simulink model "basic_complementary_filter_for_pixhawk"  (R2021b)
settings: Solver=FixedStepAuto  StartTime=0.0  StopTime=inf  RelTol=1e-3  EnableMultiTasking=on
undefined symbols (not defined in the file): DiscIntNeverNeededParam
libraries: simulink_extras x9, px4Sensorslib x3
settings Model: SimulationMode=external  ExtModeTrigDuration=10  Creator=asus  LastModifiedBy=Burhan
settings SolverCC: AlgebraicLoopSolver=TrustRegion  PositivePriorityOrder=on
settings OptimizationCC: EnhancedBackFolding=on  PassReuseOutputArgsAs=Individual arguments  MaxStackSize=64  OptimizeBlockOrder=speed  DifferentSizesBufferReuse=on  OptimizationCustomize=off  EfficientTunableParamExpr=on
settings DebuggingCC: ParameterTunabilityLossMsg=error  SFMachineParentedDataDiag=warning
settings HardwareCC: ProdBitPerPointer=32  ProdBitPerSizeT=32  ProdBitPerPtrDiffT=32  ProdLargestAtomicInteger=Long  ProdLargestAtomicFloat=Double  ProdWordSize=32  ProdLongLongMode=on  ProdHWDeviceType=ARM Compatible->ARM Cortex
settings SFSimCC: MATLABDynamicMemAlloc=off  CustomCodeUndefinedFunction=UseInterfaceOnly  SimTargetLang=C++
settings RTWCC: Description=Embedded Coder  SystemTargetFile=ert.tlc  HardwareBoard=PX4 Pixhawk Series  TLCOptions="-aInlineSetEventsForThisBaseRateFcn=TLC_FALSE -aSuppressMultiTaskScheduler=TLC_FALSE  -aRateBasedStepFcn=0"  TemplateMakefile=ert_default_tmf  GenerateReport=on  Toolchain=GNU Tools for PX4 Autopilots  IncludeHyperlinkInReport=on  LaunchReport=on  TargetLang=C++  GenerateTraceInfo=on  GenerateTraceReport=on  GenerateTraceReportSl=on  GenerateTraceReportSf=on  GenerateTraceReportEml=on
settings CodeAppCC: ForceParamTrailComments=on  IgnoreCustomStorageClasses=off  OperatorAnnotations=on  SimulinkDataObjDesc=on  SFDataObjDesc=on  InsertBlockDesc=on

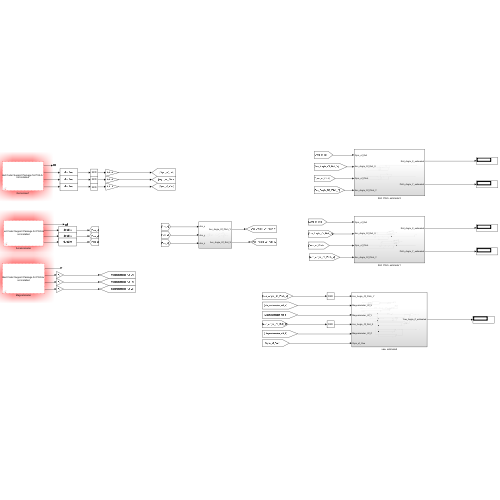
[thumbnail: Simulink's stored preview of the top-level diagram]
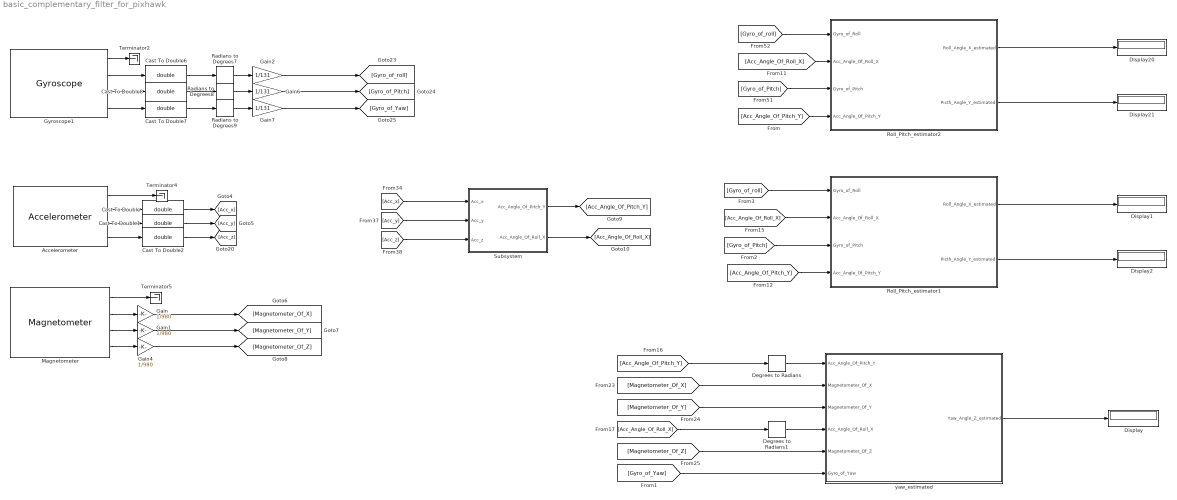
== system basic_complementary_filter_for_pixhawk ==
  Accelerometer : px4Sensorslib/Accelerometer  uorbTimeStamp=off  BlockingMode=off  BlockTimeout=1e-3  sampleTime=0.1
      settings: SourceProductName=Embedded Coder Support Package for PX4 Autopilots
  Cast To Double{,1..2,6..8} (6 alike) : DataTypeConversion  OutDataTypeStr=double
  Degrees to Radians : simulink_extras/Transformations/Degrees to Radians
  Degrees to Radians1 : simulink_extras/Transformations/Degrees to Radians
  Display{,1..2,20..21} (5 alike) : Display
  Gain : Gain  Gain=1/980
  Gain1 : Gain  Gain=1/980
  Gain2 : Gain  Gain=1/131
  Gain4 : Gain  Gain=1/980
  Gain6 : Gain  Gain=1/131
  Gain7 : Gain  Gain=1/131
  Gyroscope1 : px4Sensorslib/Gyroscope  uorbTimeStamp=off  BlockingMode=off  BlockTimeout=1e-3  sampleTime=-1
      settings: SourceProductName=Embedded Coder Support Package for PX4 Autopilots
  Magnetometer : px4Sensorslib/Magnetometer  uorbTimeStamp=off  BlockingMode=off  BlockTimeout=1e-3  sampleTime=0.1
      settings: SourceProductName=Embedded Coder Support Package for PX4 Autopilots
  Radians to Degrees7 : simulink_extras/Transformations/Radians to Degrees
  Radians to Degrees8 : simulink_extras/Transformations/Radians to Degrees
  Radians to Degrees9 : simulink_extras/Transformations/Radians to Degrees
  Roll_Pitch_estimator1 : Subsystem
  Roll_Pitch_estimator2 : Subsystem
  Subsystem : Subsystem
  Terminator2 : Terminator
  Terminator4 : Terminator
  Terminator5 : Terminator
  yaw_estimated : Subsystem
  wires:
  Cast To Double/1 -> [Acc_x]
  Accelerometer/1 -> Terminator4/1
  Accelerometer/4 -> Cast To Double2/1
  Accelerometer/2 -> Cast To Double/1
  Cast To Double6/1 -> Radians to Degrees7/1
  [Acc_Angle_Of_Pitch_Y] -> Roll_Pitch_estimator2/4(Acc_Angle_Of_Pitch_Y)
  Cast To Double7/1 -> Radians to Degrees9/1
  Roll_Pitch_estimator2/1(Roll_Angle_X_estimated) -> Display20/1
  [Gyro_of_Pitch] -> Roll_Pitch_estimator2/3(Gyro_of_Pitch)
  Gyroscope1/2 -> Cast To Double6/1
  Gyroscope1/1 -> Terminator2/1
  Gyroscope1/4 -> Cast To Double7/1
  Gain6/1 -> [Gyro_of_Pitch]
  Roll_Pitch_estimator2/2(Picth_Angle_Y_estimated) -> Display21/1
  Cast To Double1/1 -> [Acc_y]
  Accelerometer/3 -> Cast To Double1/1
  Cast To Double8/1 -> Radians to Degrees8/1
  Radians to Degrees8/1 -> Gain6/1
  Radians to Degrees7/1 -> Gain2/1
  Gyroscope1/3 -> Cast To Double8/1
  Gain7/1 -> [Gyro_of_Yaw]
  [Acc_Angle_Of_Roll_X] -> Roll_Pitch_estimator2/2(Acc_Angle_Of_Roll_X)
  Gain2/1 -> [Gyro_of_roll]
  Radians to Degrees9/1 -> Gain7/1
  [Gyro_of_roll] -> Roll_Pitch_estimator2/1(Gyro_of_Roll)
  [Gyro_of_roll] -> Roll_Pitch_estimator1/1(Gyro_of_Roll)
  [Acc_Angle_Of_Roll_X] -> Roll_Pitch_estimator1/2(Acc_Angle_Of_Roll_X)
  Roll_Pitch_estimator1/2(Picth_Angle_Y_estimated) -> Display2/1
  [Gyro_of_Pitch] -> Roll_Pitch_estimator1/3(Gyro_of_Pitch)
  Roll_Pitch_estimator1/1(Roll_Angle_X_estimated) -> Display1/1
  [Acc_Angle_Of_Pitch_Y] -> Roll_Pitch_estimator1/4(Acc_Angle_Of_Pitch_Y)
  [Acc_Angle_Of_Roll_X] -> Degrees to Radians1/1
  [Magnetometer_Of_X] -> yaw_estimated/2(Magnetometer_Of_X)
  [Magnetometer_Of_Y] -> yaw_estimated/3(Magnetometer_Of_Y)
  [Gyro_of_Yaw] -> yaw_estimated/6(Gyro_of_Yaw)
  yaw_estimated/1(Yaw_Angle_Z_estimated) -> Display/1
  [Acc_Angle_Of_Pitch_Y] -> Degrees to Radians/1
  [Magnetometer_Of_Z] -> yaw_estimated/5(Magnetometer_Of_Z)
  Magnetometer/3 -> Gain1/1
  Magnetometer/1 -> Terminator5/1
  Magnetometer/2 -> Gain/1
  Degrees to Radians/1 -> yaw_estimated/1(Acc_Angle_Of_Pitch_Y)
  Degrees to Radians1/1 -> yaw_estimated/4(Acc_Angle_Of_Roll_X)
  Cast To Double2/1 -> [Acc_z]
  Gain/1 -> [Magnetometer_Of_X]
  Gain1/1 -> [Magnetometer_Of_Y]
  Magnetometer/4 -> Gain4/1
  Gain4/1 -> [Magnetometer_Of_Z]
  [Acc_x] -> Subsystem/1(Acc_x)
  [Acc_y] -> Subsystem/2(Acc_y)
  [Acc_z] -> Subsystem/3(Acc_z)
  Subsystem/1(Acc_Angle_Of_Pitch_Y) -> [Acc_Angle_Of_Pitch_Y]
  Subsystem/2(Acc_Angle_Of_Roll_X) -> [Acc_Angle_Of_Roll_X]

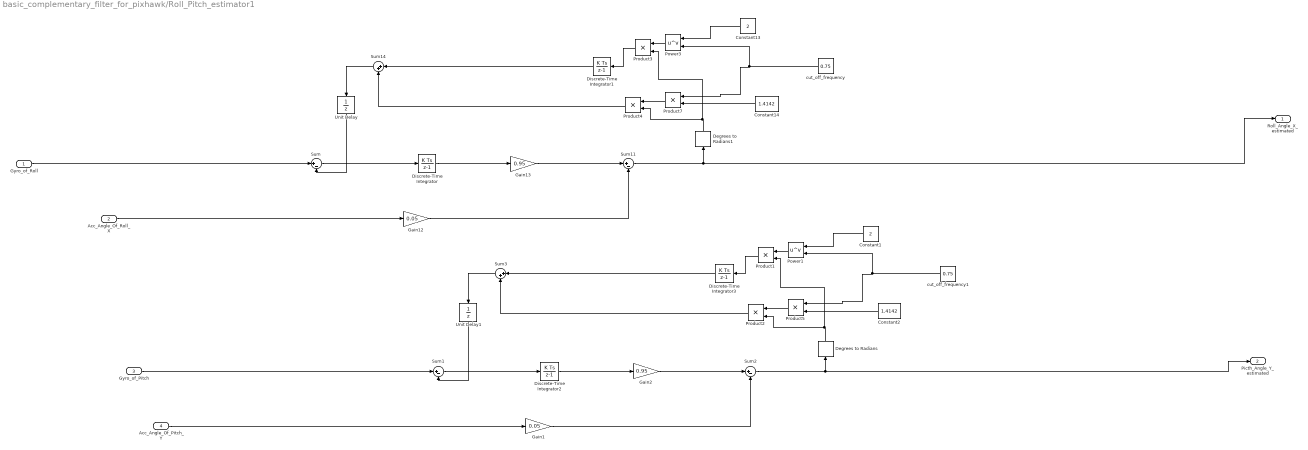
== system basic_complementary_filter_for_pixhawk/Roll_Pitch_estimator1 ==
  Gyro_of_Roll : Inport
  Acc_Angle_Of_Roll_X : Inport  Port=2
  Gyro_of_Pitch : Inport  Port=3
  Acc_Angle_Of_Pitch_Y : Inport  Port=4
  Constant1 : Constant  Value=2
  Constant13 : Constant  Value=2
  Constant14 : Constant  Value=1.4142
  Constant2 : Constant  Value=1.4142
  Degrees to Radians : simulink_extras/Transformations/Degrees to Radians
  Degrees to Radians1 : simulink_extras/Transformations/Degrees to Radians
  Discrete-Time Integrator{,1..3} (4 alike) : DiscreteIntegrator  SampleTime=-1  ICPrevOutput=DiscIntNeverNeededParam  ICPrevScaledInput=DiscIntNeverNeededParam
  Gain1 : Gain  Gain=0.05
  Gain12 : Gain  Gain=0.05
  Gain13 : Gain  Gain=0.95
  Gain2 : Gain  Gain=0.95
  Power1 : Math  Operator=pow  SignedPower=on  SaturateOnIntegerOverflow=on
  Power3 : Math  Operator=pow  SignedPower=on  SaturateOnIntegerOverflow=on
  Product{1..5,7} (6 alike) : Product
  Sum{,1..2,11} (4 alike) : Sum  Inputs=|+-
  Sum14 : Sum  Inputs=|++
  Sum3 : Sum  Inputs=|++
  Unit Delay : UnitDelay  SampleTime=-1  HasFrameUpgradeWarning=on
  Unit Delay1 : UnitDelay  SampleTime=-1  HasFrameUpgradeWarning=on
  cut_off_frequency : Constant  Value=0.75
  cut_off_frequency1 : Constant  Value=0.75
  Roll_Angle_X_estimated : Outport  VectorParamsAs1DForOutWhenUnconnected=off
  Picth_Angle_Y_estimated : Outport  Port=2  VectorParamsAs1DForOutWhenUnconnected=off
  wires:
  Discrete-Time Integrator/1 -> Gain13/1
  Acc_Angle_Of_Roll_X/1 -> Gain12/1
  Gain13/1 -> Sum11/1
  Gain12/1 -> Sum11/2
  Constant13/1 -> Power3/1
  Sum14/1 -> Unit Delay/1
  Unit Delay/1 -> Sum/2
  Discrete-Time Integrator1/1 -> Sum14/1
  Power3/1 -> Product3/1
  Constant14/1 -> Product7/2
  Product3/1 -> Discrete-Time Integrator1/1
  Product4/1 -> Sum14/2
  Product7/1 -> Product4/1
  Sum11/1 -> Degrees to Radians1/1, Roll_Angle_X_estimated/1
  Gyro_of_Roll/1 -> Sum/1
  Sum/1 -> Discrete-Time Integrator/1
  cut_off_frequency/1 -> Power3/2, Product7/1
  cut_off_frequency1/1 -> Product5/1, Power1/2
  Sum1/1 -> Discrete-Time Integrator2/1
  Gyro_of_Pitch/1 -> Sum1/1
  Sum2/1 -> Degrees to Radians/1, Picth_Angle_Y_estimated/1
  Product5/1 -> Product2/1
  Product2/1 -> Sum3/2
  Product1/1 -> Discrete-Time Integrator3/1
  Constant2/1 -> Product5/2
  Power1/1 -> Product1/1
  Discrete-Time Integrator3/1 -> Sum3/1
  Unit Delay1/1 -> Sum1/2
  Sum3/1 -> Unit Delay1/1
  Constant1/1 -> Power1/1
  Gain1/1 -> Sum2/2
  Gain2/1 -> Sum2/1
  Acc_Angle_Of_Pitch_Y/1 -> Gain1/1
  Discrete-Time Integrator2/1 -> Gain2/1
  Degrees to Radians/1 -> Product2/2, Product1/2
  Degrees to Radians1/1 -> Product3/2, Product4/2

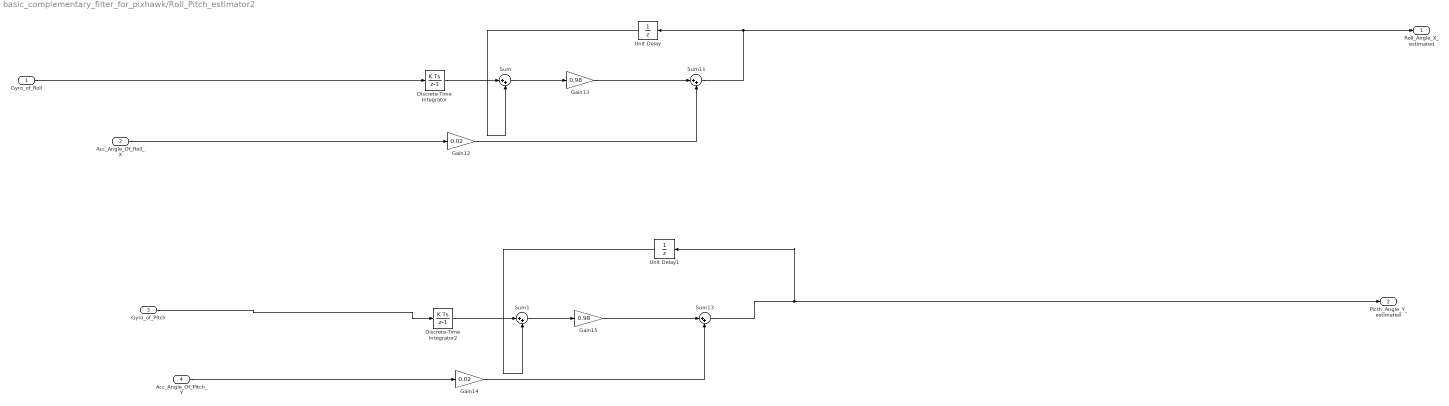
== system basic_complementary_filter_for_pixhawk/Roll_Pitch_estimator2 ==
  Gyro_of_Roll : Inport
  Acc_Angle_Of_Roll_X : Inport  Port=2
  Gyro_of_Pitch : Inport  Port=3
  Acc_Angle_Of_Pitch_Y : Inport  Port=4
  Discrete-Time Integrator : DiscreteIntegrator  SampleTime=-1  ICPrevOutput=DiscIntNeverNeededParam  ICPrevScaledInput=DiscIntNeverNeededParam
  Discrete-Time Integrator2 : DiscreteIntegrator  SampleTime=-1  ICPrevOutput=DiscIntNeverNeededParam  ICPrevScaledInput=DiscIntNeverNeededParam
  Gain12 : Gain  Gain=0.02
  Gain13 : Gain  Gain=0.98
  Gain14 : Gain  Gain=0.02
  Gain15 : Gain  Gain=0.98
  Sum{,1,11,13} (4 alike) : Sum  Inputs=|++
  Unit Delay : UnitDelay  SampleTime=-1  HasFrameUpgradeWarning=on
  Unit Delay1 : UnitDelay  SampleTime=-1  HasFrameUpgradeWarning=on
  Roll_Angle_X_estimated : Outport  VectorParamsAs1DForOutWhenUnconnected=off
  Picth_Angle_Y_estimated : Outport  Port=2  VectorParamsAs1DForOutWhenUnconnected=off
  wires:
  Sum11/1 -> Roll_Angle_X_estimated/1, Unit Delay/1
  Gyro_of_Roll/1 -> Discrete-Time Integrator/1
  Gyro_of_Pitch/1 -> Discrete-Time Integrator2/1
  Gain15/1 -> Sum13/1
  Gain12/1 -> Sum11/2
  Gain14/1 -> Sum13/2
  Gain13/1 -> Sum11/1
  Acc_Angle_Of_Pitch_Y/1 -> Gain14/1
  Sum13/1 -> Unit Delay1/1, Picth_Angle_Y_estimated/1
  Acc_Angle_Of_Roll_X/1 -> Gain12/1
  Discrete-Time Integrator/1 -> Sum/1
  Sum/1 -> Gain13/1
  Sum1/1 -> Gain15/1
  Discrete-Time Integrator2/1 -> Sum1/1
  Unit Delay/1 -> Sum/2
  Unit Delay1/1 -> Sum1/2

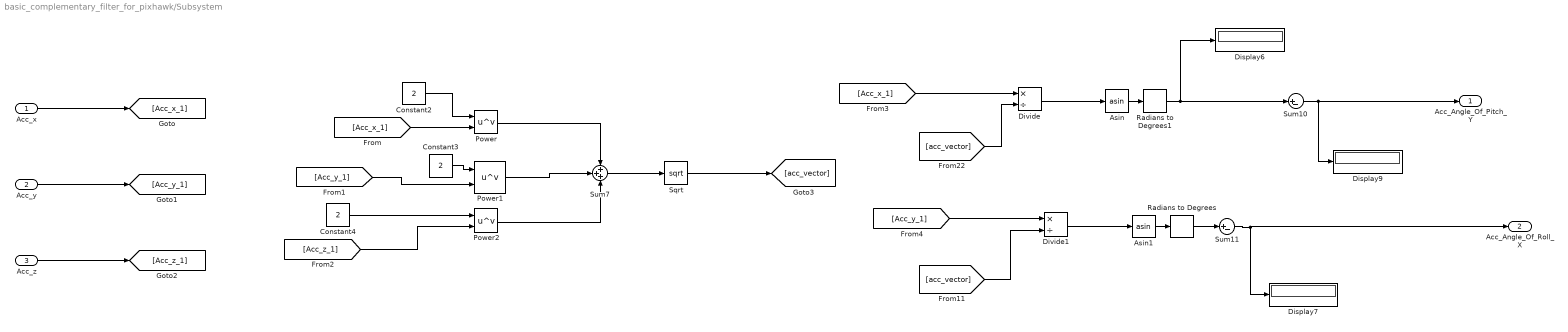
== system basic_complementary_filter_for_pixhawk/Subsystem ==
  Acc_x : Inport
  Acc_y : Inport  Port=2
  Acc_z : Inport  Port=3
  Asin : Trigonometry  Operator=asin
  Asin1 : Trigonometry  Operator=asin
  Constant2 : Constant  Value=2
  Constant3 : Constant  Value=2
  Constant4 : Constant  Value=2
  Display6 : Display
      settings: Decimation=3
  Display7 : Display
  Display9 : Display
  Divide : Product  Inputs=*/
  Divide1 : Product  Inputs=*/
  Power : Math  Operator=pow  SignedPower=on  SaturateOnIntegerOverflow=on
  Power1 : Math  Operator=pow  SignedPower=on  SaturateOnIntegerOverflow=on
  Power2 : Math  Operator=pow  SignedPower=on  SaturateOnIntegerOverflow=on
  Radians to Degrees : simulink_extras/Transformations/Radians to Degrees
  Radians to Degrees1 : simulink_extras/Transformations/Radians to Degrees
  Sqrt : Sqrt  SaturateOnIntegerOverflow=on
  Sum10 : Sum  Inputs=|+-
  Sum11 : Sum  Inputs=|+-
  Sum7 : Sum  Inputs=+++
  Acc_Angle_Of_Pitch_Y : Outport  VectorParamsAs1DForOutWhenUnconnected=off
  Acc_Angle_Of_Roll_X : Outport  Port=2  VectorParamsAs1DForOutWhenUnconnected=off
  wires:
  Divide1/1 -> Asin1/1
  Asin/1 -> Radians to Degrees1/1
  Divide/1 -> Asin/1
  Constant3/1 -> Power1/1
  Sum10/1 -> Acc_Angle_Of_Pitch_Y/1, Display9/1
  Power1/1 -> Sum7/2
  Asin1/1 -> Radians to Degrees/1
  Power/1 -> Sum7/1
  [acc_vector] -> Divide/2
  Radians to Degrees1/1 -> Sum10/1, Display6/1
  Radians to Degrees/1 -> Sum11/1
  Power2/1 -> Sum7/3
  Constant4/1 -> Power2/1
  Constant2/1 -> Power/1
  [acc_vector] -> Divide1/2
  Sqrt/1 -> [acc_vector]
  Sum11/1 -> Acc_Angle_Of_Roll_X/1, Display7/1
  [Acc_x_1] -> Divide/1
  [Acc_y_1] -> Divide1/1
  Sum7/1 -> Sqrt/1
  Acc_x/1 -> [Acc_x_1]
  Acc_y/1 -> [Acc_y_1]
  Acc_z/1 -> [Acc_z_1]
  [Acc_x_1] -> Power/2
  [Acc_y_1] -> Power1/2
  [Acc_z_1] -> Power2/2

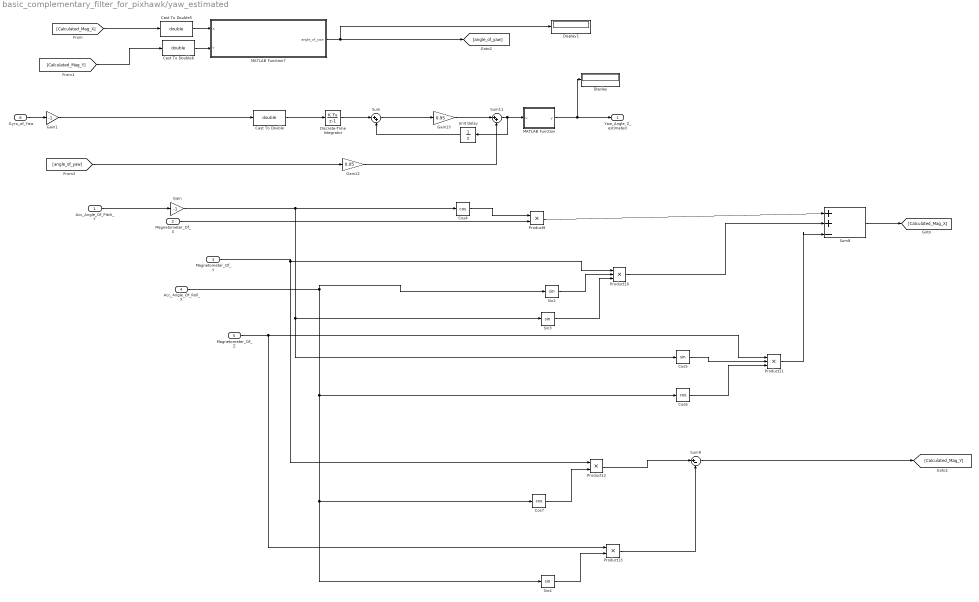
== system basic_complementary_filter_for_pixhawk/yaw_estimated ==
  Acc_Angle_Of_Pitch_Y : Inport
  Magnetometer_Of_X : Inport  Port=2
  Magnetometer_Of_Y : Inport  Port=3
  Acc_Angle_Of_Roll_X : Inport  Port=4
  Magnetometer_Of_Z : Inport  Port=5
  Gyro_of_Yaw : Inport  Port=6
  Cast To Double : DataTypeConversion  OutDataTypeStr=double
  Cast To Double5 : DataTypeConversion  OutDataTypeStr=double
  Cast To Double6 : DataTypeConversion  OutDataTypeStr=double
  Cos4 : Trigonometry  Operator=cos
  Cos5 : Trigonometry
  Cos6 : Trigonometry  Operator=cos
  Cos7 : Trigonometry  Operator=cos
  Discrete-Time Integrator : DiscreteIntegrator  SampleTime=-1  ICPrevOutput=DiscIntNeverNeededParam  ICPrevScaledInput=DiscIntNeverNeededParam
  Display : Display
  Display1 : Display
  Gain : Gain  Gain=-1
  Gain1 : Gain  Gain=-1
  Gain12 : Gain  Gain=0.05
  Gain13 : Gain  Gain=0.95
  MATLAB Function : MATLAB Function  TreatAsAtomicUnit=on
  MATLAB Function7 : MATLAB Function  TreatAsAtomicUnit=on
  Product10 : Product  Inputs=3
  Product11 : Product  Inputs=3
  Product12 : Product
  Product13 : Product
  Product9 : Product
  Sin2 : Trigonometry
  Sin3 : Trigonometry
  Sin4 : Trigonometry
  Sum : Sum  Inputs=|++
  Sum11 : Sum  Inputs=|++
  Sum8 : Sum  Inputs=|++-
  Sum9 : Sum  Inputs=|+-
  Unit Delay : UnitDelay  SampleTime=-1  HasFrameUpgradeWarning=on
  Yaw_Angle_Z_estimated : Outport  VectorParamsAs1DForOutWhenUnconnected=off
  wires:
  Acc_Angle_Of_Roll_X/1 -> Sin4/1, Cos7/1, Cos6/1, Sin2/1
  Cos6/1 -> Product11/3
  Product11/1 -> Sum8/3
  [Calculated_Mag_X] -> Cast To Double5/1
  Acc_Angle_Of_Pitch_Y/1 -> Gain/1
  Magnetometer_Of_X/1 -> Product9/2
  Magnetometer_Of_Y/1 -> Product12/1, Product10/1
  Sin2/1 -> Product10/2
  Product12/1 -> Sum9/1
  Sin3/1 -> Product10/3
  Cos7/1 -> Product12/2
  Cos5/1 -> Product11/2
  Sin4/1 -> Product13/2
  Product9/1 -> Sum8/1
  Product10/1 -> Sum8/2
  Cast To Double5/1 -> MATLAB Function7/1(X)
  Product13/1 -> Sum9/2
  Magnetometer_Of_Z/1 -> Product13/1, Product11/1
  Cast To Double6/1 -> MATLAB Function7/2(Y)
  [Calculated_Mag_Y] -> Cast To Double6/1
  Sum9/1 -> [Calculated_Mag_Y]
  Cos4/1 -> Product9/1
  Sum8/1 -> [Calculated_Mag_X]
  [angle_of_yaw] -> Gain12/1
  Gyro_of_Yaw/1 -> Gain1/1
  Cast To Double/1 -> Discrete-Time Integrator/1
  Gain12/1 -> Sum11/2
  Gain13/1 -> Sum11/1
  Sum11/1 -> Unit Delay/1, MATLAB Function/1(u)
  MATLAB Function7/1(angle_of_yaw) -> Display1/1, [angle_of_yaw]
  Discrete-Time Integrator/1 -> Sum/1
  Sum/1 -> Gain13/1
  Unit Delay/1 -> Sum/2
  Gain/1 -> Cos5/1, Sin3/1, Cos4/1
  Gain1/1 -> Cast To Double/1
  MATLAB Function/1(y) -> Display/1, Yaw_Angle_Z_estimated/1

== matlab function basic_complementary_filter_for_pixhawk/yaw_estimated/MATLAB Function7 ==
  data: X input; angle_of_yaw output; Y input
function angle_of_yaw = fcn(X, Y)

if Y < 0
    angle_of_yaw = 180+(180+(atan2(Y,X)* 180/pi))
else
    angle_of_yaw = atan2(Y,X)*180/pi
end

angle_of_yaw= angle_of_yaw-57;


end

== matlab function basic_complementary_filter_for_pixhawk/yaw_estimated/MATLAB Function ==
  data: u input; y output
function y = fcn(u)
if u < 0
    y = u + 360
elseif u > 360
    y = u - 360
else
    y = u
end
end
